simulink model "PWM_Simulation"  (R2016a)
settings: Solver=ode4  StartTime=0.0  StopTime=0.1  FixedStep=1e-5  RelTol=1e-3
libraries: simulink x1
settings Model: Creator=admin  LastModifiedBy=admin

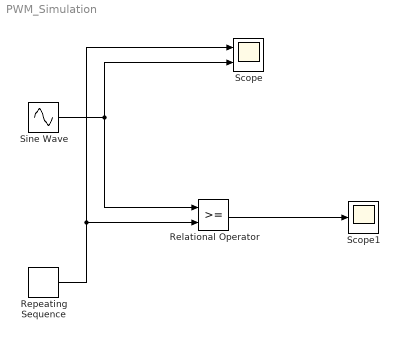
== system PWM_Simulation ==
  Relational Operator : RelationalOperator  OutDataTypeStr=boolean
  Repeating Sequence : simulink/Sources/Repeating Sequence  rep_seq_t=[0 1 2]*[1/100]  rep_seq_y=[0 1 0]
  Scope : Scope  NumInputPorts=2
  Scope1 : Scope
  Sine Wave : Sin  Frequency=2*pi*25  SampleTime=0
  wires:
  Sine Wave/1 -> Relational Operator/1, Scope/2
  Repeating Sequence/1 -> Relational Operator/2, Scope/1
  Relational Operator/1 -> Scope1/1
